simulink library "int_node_maker"  (R2018b)
settings: Solver=VariableStepAuto  StartTime=0.0  StopTime=10.0  RelTol=1e-3
values from neighbouring files (symbols this model uses):
  N = 5    [test_fn.m]
  R1_o = [   -2.5000 ... (first row only)    [test_fn.m]
  Rn_o = [   -2.5271 ... (first row only)    [test_fn.m]
settings Model: Creator=Ayaz  LastModifiedBy=Ayaz

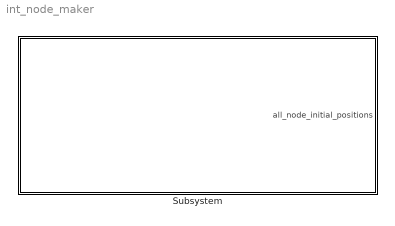
== system int_node_maker ==
  Subsystem : Subsystem  mask{N=N, R1_o=R1_o, Rn_o=Rn_o}
      mask prompts: N "Number of nodes"; R1_o "First node initial position vector"; Rn_o "Last node initial position vector"

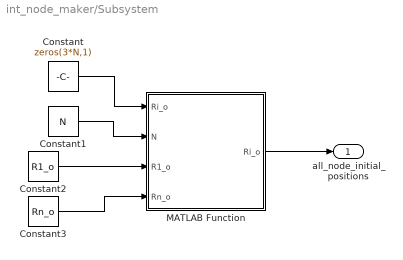
== system int_node_maker/Subsystem ==
  Constant : Constant  Value=zeros(3*N,1)
  Constant1 : Constant  Value=N
  Constant2 : Constant  Value=R1_o
  Constant3 : Constant  Value=Rn_o
  MATLAB Function : MATLAB Function  TreatAsAtomicUnit=on
  all_node_initial_positions : Outport
  wires:
  MATLAB Function/1(Ri_o) -> all_node_initial_positions/1
  Constant2/1 -> MATLAB Function/3(R1_o)
  Constant3/1 -> MATLAB Function/4(Rn_o)
  Constant/1 -> MATLAB Function/1("Ri_o ")
  Constant1/1 -> MATLAB Function/2(N)

== matlab function int_node_maker/Subsystem/MATLAB Function ==
  data: Ri_o input; N input; Ri_o output; R1_o input; Rn_o input
function Ri_o = fcn(Ri_o,N,R1_o,Rn_o)


for i = 1:N
    
    if i == 1
        Ri_o((3*i-2):(3*i),1) = R1_o;
        
    elseif i>1 && i<N
        Ri_o((3*i-2):(3*i),1) = R1_o + ((Rn_o - R1_o)*(i-1)/(N-1));
        
    elseif i == N
        Ri_o((3*i-2):(3*i),1) = Rn_o;
   
    end
end

end
